simulink model "OM2"  (R2015b)
settings: Solver=VariableStepAuto  SolverMode=SingleTasking  StartTime=0.0  StopTime=t_final  MaxStep=0.001  RelTol=1e-3
undefined symbols (not defined in the file): K1, K2, Kd, Ki, Kia, Kp, Kpa, st, T0, T1, T2, Tur, Tzap
settings Model: Creator=Anton Mayorov  LastModifiedBy=bedla
settings DataIOCC: LimitDataPoints=off
settings DebuggingCC: AllowSymbolicDim=on  SFUnexpectedBacktrackingDiag=error  SFNoUnconditionalDefaultTransitionDiag=error
settings ModelReferenceCC: PropagateSignalLabelsOutOfModel=on
settings GRTTargetCC: TargetLangStandard=C99 (ISO)
settings ConfigComp: CovMetricSettings=dwe  CovHtmlReporting=off  CovSaveCumulativeToWorkspaceVar=off  CovSaveSingleToWorkspaceVar=off  CovModelRefEnable=Off  CovExternalEMLEnable=on

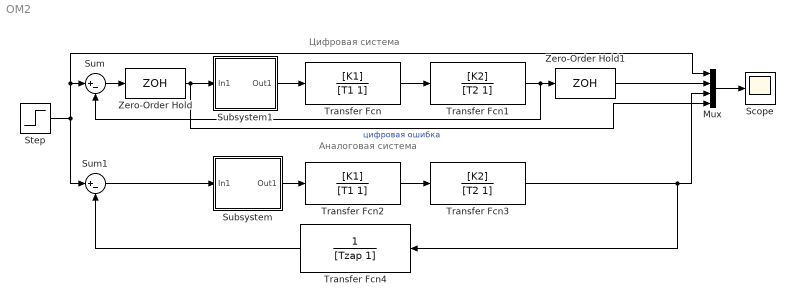
== system OM2 ==
  note: Аналоговая система
  note: Цифровая система
  Mux : Mux
  Scope : Scope
  Step : Step  Time=st  SampleTime=0
  Subsystem : Subsystem
  Subsystem1 : Subsystem
  Sum : Sum  Inputs=|+-
  Sum1 : Sum  Inputs=|+-
  Transfer Fcn : TransferFcn  Numerator=[K1]  Denominator=[T1 1]
  Transfer Fcn1 : TransferFcn  Numerator=[K2]  Denominator=[T2 1]
  Transfer Fcn2 : TransferFcn  Numerator=[K1]  Denominator=[T1 1]
  Transfer Fcn3 : TransferFcn  Numerator=[K2]  Denominator=[T2 1]
  Transfer Fcn4 : TransferFcn  Denominator=[Tzap 1]
  Zero-Order Hold : ZeroOrderHold  SampleTime=T0
  Zero-Order Hold1 : ZeroOrderHold  SampleTime=T0
  wires:
  Zero-Order Hold/1 -> Subsystem1/1(In1), Mux/4  "цифровая ошибка"
  Transfer Fcn/1 -> Transfer Fcn1/1
  Mux/1 -> Scope/1
  Subsystem1/1(Out1) -> Transfer Fcn/1
  Transfer Fcn1/1 -> Sum/2, Zero-Order Hold1/1
  Sum/1 -> Zero-Order Hold/1
  Step/1 -> Mux/1, Sum/1, Sum1/1
  Sum1/1 -> Subsystem/1(In1)
  Transfer Fcn3/1 -> Mux/3, Transfer Fcn4/1
  Subsystem/1(Out1) -> Transfer Fcn2/1
  Transfer Fcn2/1 -> Transfer Fcn3/1
  Zero-Order Hold1/1 -> Mux/2
  Transfer Fcn4/1 -> Sum1/2

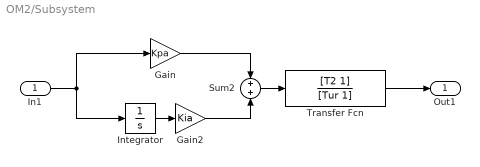
== system OM2/Subsystem ==
  In1 : Inport
  Gain : Gain  Gain=Kpa
  Gain2 : Gain  Gain=Kia
  Integrator : Integrator
  Sum2 : Sum
  Transfer Fcn : TransferFcn  Numerator=[T2 1]  Denominator=[Tur 1]
  Out1 : Outport
  wires:
  In1/1 -> Gain/1, Integrator/1
  Integrator/1 -> Gain2/1
  Gain/1 -> Sum2/1
  Sum2/1 -> Transfer Fcn/1
  Gain2/1 -> Sum2/2
  Transfer Fcn/1 -> Out1/1

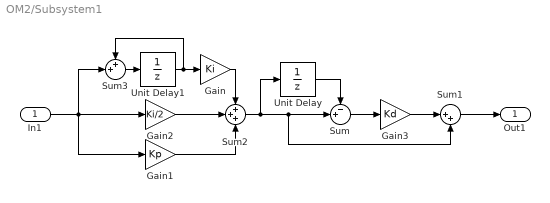
== system OM2/Subsystem1 ==
  In1 : Inport
  Gain : Gain  Gain=Ki
  Gain1 : Gain  Gain=Kp
  Gain2 : Gain  Gain=Ki/2
  Gain3 : Gain  Gain=Kd
  Sum : Sum  Inputs=-+|
  Sum1 : Sum  Inputs=|++
  Sum2 : Sum  Inputs=+++
  Sum3 : Sum  Inputs=++|
  Unit Delay : UnitDelay  SampleTime=T0  HasFrameUpgradeWarning=on
  Unit Delay1 : UnitDelay  SampleTime=-1  HasFrameUpgradeWarning=on
  Out1 : Outport
  wires:
  Sum3/1 -> Unit Delay1/1
  Unit Delay1/1 -> Gain/1, Sum3/1
  Gain/1 -> Sum2/1
  In1/1 -> Gain2/1, Gain1/1, Sum3/2
  Gain2/1 -> Sum2/2
  Gain1/1 -> Sum2/3
  Gain3/1 -> Sum1/1
  Sum/1 -> Gain3/1
  Sum2/1 -> Sum1/2, Sum/2, Unit Delay/1
  Unit Delay/1 -> Sum/1
  Sum1/1 -> Out1/1
